simulink model "TestDeriveMatlabFun"  (R2013b)
settings: Solver=ode45  StartTime=0.0  StopTime=10.0  RelTol=1e-3
settings Model: Creator=Think79  LastModifiedBy=Think79

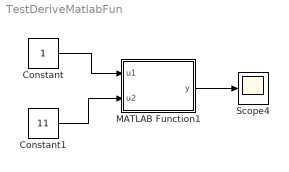
== system TestDeriveMatlabFun ==
  Constant : Constant
  Constant1 : Constant  Value=11
  MATLAB Function1 : MATLAB Function  TreatAsAtomicUnit=on
  Scope4 : Scope
      settings: YMin=-2.25  YMax=0.75
  wires:
  Constant/1 -> MATLAB Function1/1(u1)
  Constant1/1 -> MATLAB Function1/2(u2)
  MATLAB Function1/1(y) -> Scope4/1

== matlab function TestDeriveMatlabFun/MATLAB Function1 ==
  data: u1 input; y output; u2 input
function y = fcn(u1,u2)
%#codegen

if u2>22.5
    theta=45-u2;
else
    theta=u2;
end


FluxLine20=0:0.08:0.08*19; 
thetaRow001=0:0.01:22.5;    % theta 0.01
thetaRow50=thetaRow001(1:45:2250);  % theta row 50
DeriveThetaofWrow50line20=[0.0000 	0.0005 	0.0018 	0.0041 	0.0073 	0.0114 	0.0165 	0.0224 	0.0290 	0.0367 	0.0456 	0.0551 	0.0648 	0.0747 	0.0853 	0.0953 	0.1031 	0.1079 	0.1097 	0.1088 
0.0000 	0.0015 	0.0060 	0.0135 	0.0240 	0.0374 	0.0539 	0.0733 	0.0956 	0.1210 	0.1496 	0.1809 	0.2141 	0.2510 	0.2926 	0.3343 	0.3704 	0.3976 	0.4149 	0.4238 
0.0000 	0.0026 	0.0103 	0.0232 	0.0413 	0.0645 	0.0928 	0.1264 	0.1650 	0.2087 	0.2580 	0.3117 	0.3688 	0.4323 	0.5047 	0.5785 	0.6434 	0.6935 	0.7264 	0.7443 
0.0000 	0.0037 	0.0148 	0.0334 	0.0593 	0.0927 	0.1333 	0.1815 	0.2371 	0.3000 	0.3706 	0.4476 	0.5289 	0.6186 	0.7215 	0.8279 	0.9222 	0.9955 	1.0441 	1.0705 
0.0000 	0.0050 	0.0199 	0.0449 	0.0797 	0.1246 	0.1793 	0.2441 	0.3189 	0.4035 	0.4983 	0.6015 	0.7099 	0.8278 	0.9633 	1.1058 	1.2341 	1.3350 	1.4030 	1.4403 
0.0000 	0.0066 	0.0264 	0.0595 	0.1057 	0.1652 	0.2376 	0.3238 	0.4230 	0.5347 	0.6599 	0.7967 	0.9394 	1.0913 	1.2657 	1.4535 	1.6273 	1.7677 	1.8654 	1.9210 
0.0000 	0.0079 	0.0315 	0.0709 	0.1260 	0.1970 	0.2835 	0.3865 	0.5050 	0.6384 	0.7873 	0.9488 	1.1161 	1.2923 	1.4945 	1.7168 	1.9266 	2.0974 	2.2166 	2.2839 
0.0000 	0.0087 	0.0349 	0.0786 	0.1398 	0.2184 	0.3145 	0.4287 	0.5604 	0.7090 	0.8735 	1.0494 	1.2300 	1.4179 	1.6333 	1.8758 	2.1087 	2.2968 	2.4242 	2.4912 
0.0000 	0.0102 	0.0408 	0.0919 	0.1633 	0.2552 	0.3675 	0.5004 	0.6532 	0.8257 	1.0173 	1.2224 	1.4297 	1.6363 	1.8676 	2.1390 	2.4083 	2.6227 	2.7591 	2.8197 
0.0000 	0.0121 	0.0483 	0.1086 	0.1932 	0.3018 	0.4347 	0.5911 	0.7714 	0.9736 	1.1950 	1.4318 	1.6728 	1.9077 	2.1570 	2.4492 	2.7488 	2.9930 	3.1505 	3.2195 
0.0000 	0.0140 	0.0559 	0.1258 	0.2237 	0.3495 	0.5034 	0.6841 	0.8938 	1.1262 	1.3704 	1.6280 	1.8994 	2.1702 	2.4355 	2.7243 	3.0299 	3.3001 	3.4975 	3.6057 
0.0000 	0.0156 	0.0622 	0.1400 	0.2490 	0.3890 	0.5602 	0.7614 	0.9923 	1.2457 	1.5107 	1.7853 	2.0700 	2.3537 	2.6223 	2.9047 	3.2166 	3.5121 	3.7448 	3.8896 
0.0000 	0.0170 	0.0679 	0.1527 	0.2715 	0.4242 	0.6106 	0.8301 	1.0765 	1.3427 	1.6233 	1.9097 	2.1955 	2.4765 	2.7456 	3.0289 	3.3526 	3.6737 	3.9341 	4.1050 
0.0000 	0.0187 	0.0747 	0.1681 	0.2988 	0.4668 	0.6720 	0.9122 	1.1778 	1.4553 	1.7376 	2.0262 	2.3160 	2.6068 	2.8982 	3.1991 	3.5391 	3.8868 	4.1721 	4.3585 
0.0000 	0.0206 	0.0824 	0.1855 	0.3297 	0.5151 	0.7408 	1.0011 	1.2830 	1.5708 	1.8582 	2.1465 	2.4373 	2.7384 	3.0530 	3.3758 	3.7294 	4.0966 	4.4059 	4.6121 
0.0000 	0.0223 	0.0892 	0.2007 	0.3569 	0.5574 	0.8001 	1.0746 	1.3638 	1.6577 	1.9547 	2.2426 	2.5303 	2.8366 	3.1639 	3.5028 	3.8636 	4.2419 	4.5753 	4.8085 
0.0000 	0.0221 	0.0883 	0.1988 	0.3534 	0.5518 	0.7906 	1.0570 	1.3344 	1.6173 	1.9009 	2.1832 	2.4731 	2.7787 	3.1033 	3.4377 	3.7974 	4.1891 	4.5462 	4.7967 
0.0000 	0.0191 	0.0764 	0.1718 	0.3055 	0.4771 	0.6842 	0.9192 	1.1716 	1.4363 	1.7044 	1.9844 	2.2824 	2.5927 	2.9143 	3.2422 	3.5991 	4.0025 	4.3835 	4.6497 
0.0000 	0.0133 	0.0532 	0.1196 	0.2127 	0.3326 	0.4814 	0.6665 	0.8885 	1.1393 	1.4109 	1.6993 	2.0096 	2.3376 	2.6701 	3.0079 	3.3662 	3.7745 	4.1789 	4.4688 
0.0000 	0.0102 	0.0406 	0.0914 	0.1624 	0.2542 	0.3703 	0.5232 	0.7247 	0.9702 	1.2472 	1.5436 	1.8597 	2.1949 	2.5413 	2.8959 	3.2550 	3.6583 	4.0784 	4.4015 
0.0000 	0.0096 	0.0385 	0.0866 	0.1539 	0.2407 	0.3491 	0.4877 	0.6748 	0.9152 	1.1923 	1.4918 	1.8058 	2.1360 	2.4895 	2.8578 	3.2189 	3.6109 	4.0375 	4.3970 
0.0000 	0.0091 	0.0363 	0.0816 	0.1451 	0.2268 	0.3276 	0.4537 	0.6187 	0.8356 	1.1017 	1.3959 	1.7028 	2.0238 	2.3627 	2.7271 	3.0965 	3.4807 	3.9044 	4.2902 
0.0000 	0.0091 	0.0363 	0.0817 	0.1453 	0.2269 	0.3271 	0.4491 	0.6022 	0.8003 	1.0520 	1.3379 	1.6391 	1.9552 	2.2798 	2.6280 	2.9996 	3.3814 	3.8020 	4.2112 
0.0000 	0.0095 	0.0378 	0.0851 	0.1512 	0.2363 	0.3405 	0.4644 	0.6162 	0.8051 	1.0407 	1.3174 	1.6165 	1.9328 	2.2527 	2.5812 	2.9452 	3.3281 	3.7489 	4.1805 
0.0000 	0.0083 	0.0330 	0.0743 	0.1321 	0.2065 	0.2975 	0.4056 	0.5357 	0.6997 	0.9101 	1.1741 	1.4703 	1.7800 	2.1014 	2.4307 	2.7866 	3.1623 	3.5840 	4.0306 
0.0000 	0.0064 	0.0257 	0.0578 	0.1027 	0.1606 	0.2313 	0.3160 	0.4165 	0.5471 	0.7235 	0.9608 	1.2443 	1.5428 	1.8622 	2.1998 	2.5535 	2.9241 	3.3459 	3.8004 
0.0000 	0.0051 	0.0202 	0.0454 	0.0807 	0.1261 	0.1817 	0.2479 	0.3264 	0.4257 	0.5622 	0.7533 	1.0068 	1.2933 	1.6000 	1.9385 	2.2990 	2.6766 	3.0963 	3.5527 
0.0000 	0.0044 	0.0176 	0.0395 	0.0701 	0.1096 	0.1578 	0.2150 	0.2826 	0.3647 	0.4753 	0.6318 	0.8520 	1.1244 	1.4250 	1.7558 	2.1167 	2.5006 	2.9149 	3.3681 
0.0000 	0.0043 	0.0171 	0.0384 	0.0682 	0.1066 	0.1535 	0.2091 	0.2741 	0.3513 	0.4496 	0.5853 	0.7741 	1.0275 	1.3237 	1.6420 	1.9949 	2.3790 	2.7848 	3.2292 
0.0000 	0.0042 	0.0169 	0.0380 	0.0676 	0.1055 	0.1520 	0.2069 	0.2707 	0.3453 	0.4357 	0.5542 	0.7172 	0.9413 	1.2176 	1.5267 	1.8670 	2.2402 	2.6353 	3.0645 
0.0000 	0.0040 	0.0161 	0.0362 	0.0644 	0.1006 	0.1449 	0.1972 	0.2577 	0.3276 	0.4099 	0.5130 	0.6524 	0.8432 	1.0919 	1.3856 	1.7117 	2.0706 	2.4538 	2.8728 
0.0000 	0.0036 	0.0145 	0.0327 	0.0581 	0.0907 	0.1306 	0.1779 	0.2323 	0.2947 	0.3675 	0.4567 	0.5734 	0.7320 	0.9501 	1.2194 	1.5308 	1.8758 	2.2475 	2.6633 
0.0000 	0.0033 	0.0131 	0.0295 	0.0524 	0.0819 	0.1178 	0.1605 	0.2097 	0.2658 	0.3303 	0.4079 	0.5068 	0.6419 	0.8283 	1.0715 	1.3675 	1.6997 	2.0640 	2.4709 
0.0000 	0.0029 	0.0116 	0.0261 	0.0464 	0.0725 	0.1044 	0.1421 	0.1858 	0.2353 	0.2918 	0.3583 	0.4416 	0.5556 	0.7110 	0.9247 	1.1996 	1.5196 	1.8777 	2.2734 
0.0000 	0.0024 	0.0098 	0.0220 	0.0391 	0.0611 	0.0880 	0.1198 	0.1566 	0.1983 	0.2456 	0.3003 	0.3680 	0.4575 	0.5849 	0.7641 	1.0081 	1.3155 	1.6653 	2.0518 
0.0000 	0.0021 	0.0084 	0.0189 	0.0337 	0.0526 	0.0757 	0.1031 	0.1347 	0.1707 	0.2113 	0.2575 	0.3139 	0.3869 	0.4924 	0.6416 	0.8532 	1.1394 	1.4785 	1.8585 
0.0000 	0.0020 	0.0081 	0.0181 	0.0323 	0.0504 	0.0725 	0.0987 	0.1290 	0.1634 	0.2021 	0.2461 	0.2981 	0.3649 	0.4571 	0.5862 	0.7710 	1.0299 	1.3553 	1.7299 
0.0000 	0.0023 	0.0093 	0.0210 	0.0374 	0.0584 	0.0841 	0.1144 	0.1494 	0.1890 	0.2336 	0.2846 	0.3423 	0.4117 	0.5019 	0.6268 	0.7993 	1.0338 	1.3415 	1.7076 
0.0000 	0.0024 	0.0098 	0.0220 	0.0391 	0.0611 	0.0880 	0.1198 	0.1565 	0.1977 	0.2439 	0.2968 	0.3565 	0.4243 	0.5078 	0.6207 	0.7736 	0.9772 	1.2521 	1.5928 
0.0000 	0.0021 	0.0085 	0.0191 	0.0340 	0.0531 	0.0765 	0.1043 	0.1363 	0.1720 	0.2115 	0.2564 	0.3091 	0.3669 	0.4338 	0.5213 	0.6416 	0.8070 	1.0337 	1.3309 
0.0000 	0.0017 	0.0067 	0.0151 	0.0268 	0.0418 	0.0602 	0.0821 	0.1075 	0.1357 	0.1666 	0.2012 	0.2425 	0.2892 	0.3409 	0.4076 	0.5030 	0.6354 	0.8193 	1.0765 
0.0000 	0.0014 	0.0056 	0.0125 	0.0223 	0.0348 	0.0500 	0.0682 	0.0894 	0.1132 	0.1391 	0.1672 	0.2002 	0.2404 	0.2843 	0.3390 	0.4178 	0.5263 	0.6778 	0.8987 
0.0000 	0.0015 	0.0060 	0.0134 	0.0238 	0.0372 	0.0536 	0.0730 	0.0957 	0.1214 	0.1495 	0.1793 	0.2129 	0.2543 	0.3011 	0.3538 	0.4226 	0.5178 	0.6490 	0.8355 
0.0000 	0.0015 	0.0061 	0.0138 	0.0246 	0.0384 	0.0553 	0.0752 	0.0984 	0.1251 	0.1548 	0.1862 	0.2196 	0.2595 	0.3070 	0.3582 	0.4191 	0.5034 	0.6167 	0.7721 
0.0000 	0.0014 	0.0058 	0.0130 	0.0233 	0.0365 	0.0525 	0.0712 	0.0929 	0.1181 	0.1469 	0.1779 	0.2094 	0.2441 	0.2878 	0.3355 	0.3895 	0.4620 	0.5567 	0.6839 
0.0000 	0.0013 	0.0051 	0.0115 	0.0206 	0.0323 	0.0466 	0.0631 	0.0820 	0.1040 	0.1297 	0.1584 	0.1873 	0.2169 	0.2532 	0.2948 	0.3419 	0.3995 	0.4734 	0.5726 
0.0000 	0.0009 	0.0034 	0.0077 	0.0139 	0.0218 	0.0315 	0.0426 	0.0553 	0.0699 	0.0873 	0.1072 	0.1275 	0.1471 	0.1703 	0.1982 	0.2305 	0.2677 	0.3153 	0.3811 
0.0000 	0.0002 	0.0010 	0.0022 	0.0039 	0.0061 	0.0088 	0.0119 	0.0154 	0.0195 	0.0243 	0.0300 	0.0359 	0.0414 	0.0477 	0.0558 	0.0659 	0.0789 	0.0972 	0.1257 
0.0000 	-0.0001 	-0.0004 	-0.0009 	-0.0017 	-0.0026 	-0.0037 	-0.0051 	-0.0066 	-0.0084 	-0.0104 	-0.0127 	-0.0150 	-0.0173 	-0.0203 	-0.0233 	-0.0260 	-0.0275 	-0.0277 	-0.0239 
0.0000 	-0.0001 	-0.0005 	-0.0011 	-0.0019 	-0.0030 	-0.0044 	-0.0059 	-0.0077 	-0.0097 	-0.0120 	-0.0148 	-0.0177 	-0.0205 	-0.0237 	-0.0276 	-0.0322 	-0.0373 	-0.0436 	-0.0501 
];

if u1<=0
    y=0;
else
    y=interp2(FluxLine20,thetaRow50,DeriveThetaofWrow50line20,1,14,'spline');
end
end
